simulink library "common_lib"  (R2023a)
settings: Solver=ode45  StartTime=0.0  StopTime=10.0  RelTol=1e-3
undefined symbols (not defined in the file): ACCEL_PRE_MULT, APDT_SrvcMgr_IRVHVDCSubFcnReq, C_C1GearNumbers, C_C1GearRatios, C_Calibration, C_DitherWaveform, C_GearOffset, C_GearRatioIn, C_GearRatioInverseOut, C_GearRatioOut, CLUTCH_INNER_LOOP_UPDATE_RATE, CONSTANT, DEGRADED_MODE_SIZE, Dem_EventStatusType, DiscIntNeverNeededParam, F_FAULT_ENUM, F_NOFAULT, F_OUTOFRANGE, F_RATELIMIT, FALSE, FMI14_SPECIAL_INSTRUCTIONS, FMI20_DATA_DRIFTED_HIGH, FMI21_DATA_DRIFTED_LOW, FMI29_RESERVED_FOR_SAE_ASSIGNMENT, FMI30_RESERVED_FOR_SAE_ASSIGNMENT, FMI31_CONDITION_EXISTS, FMI32_NO_FAULT, IC, k_accel, k_mean, MAX_UINT32, MEAN_PRE_MULT, NTriggers, QLTY_SIGNAL_FAILED, QLTY_SIGNAL_FULLY_FUNCTION, QLTY_SIGNAL_SUBSTITUTED_BY_1ST_CHOICE, QLTY_SIGNAL_SUBSTITUTED_BY_2ND_CHOICE, QLTY_SIGNAL_SUBSTITUTED_BY_3RD_CHOICE, QLTY_SIGNAL_SUBSTITUTED_BY_4TH_CHOICE, SAMPLE_TIME_100us, SAMPLETIME_10ms_Int, SATURATION_U16, simin, T_TestPoint, TF_FALSE, TF_TRUE, TimeStep, TRUE, WORKSPACE_UPDATE_RATE, ZERO, Zero
libraries: $bdroot x123, simulink x28, simulink_extras x4, MBD_EPS_Local_Blockset x4
(part 4 of 10)

== system common_lib/Approved Simulink/Basic IO ==
  note: HWin/ HWout
  note: Product Test
  note: Data Monitor, VPA, SnapShot
  Inport : Inport
  C_Calibration : $bdroot/IO/Calibration with Pretty Print Value  CalValue=C_Calibration  scaling=None
  Constant : Constant  Value=CONSTANT  SampleTime=-1
  DRDataStoreRead : DataStoreRead  DataStoreName=DataStoreRead  SampleTime=0  IndexOptions=Index vector (dialog)  Indices=1  OutputSizes=1
  DRDataStoreRead1 : DataStoreRead  DataStoreName=PT_ProductTest_Read  SampleTime=0  IndexOptions=Index vector (dialog)  Indices=1  OutputSizes=1
  DRDataStoreRead2 : DataStoreRead  DataStoreName=DM_DataMonitor_Read  SampleTime=0  IndexOptions=Index vector (dialog)  Indices=1  OutputSizes=1
  DSDataStoreMemory : DataStoreMemory  DataStoreName=DataStoreMemory  ShowAdditionalParam=off
  DSDataStoreMemory1 : DataStoreMemory  DataStoreName=PT_ProductTest_Memory  ShowAdditionalParam=off
  DSDataStoreMemory2 : DataStoreMemory  DataStoreName=DM_DataMonitor  ShowAdditionalParam=off
  DWDataStoreWrite : DataStoreWrite  DataStoreName=DataStoreWrite  IndexOptions=Index vector (dialog)  Indices=1  OutputSizes=1
  DWDataStoreWrite1 : DataStoreWrite  DataStoreName=DataStoreWrite  IndexOptions=Index vector (dialog)  Indices=1  OutputSizes=1
  DWDataStoreWrite2 : DataStoreWrite  DataStoreName=DM_DataMonitor_Write  IndexOptions=Index vector (dialog)  Indices=1  OutputSizes=1
  Ground : Ground
  M_MonitorParameter : ToWorkspace  VariableName=MonitorParameter  SampleTime=WORKSPACE_UPDATE_RATE
      settings: Decimation=WORKSPACE_DECIMATION
  M_MonitorParameter1 : Subsystem  mask{work=ToWorkspace}
      mask prompts: work "Variable Name"
      mask init:
      | set_param([gcb,'/towork'],'VariableName',work);
      | a = get_param([gcb '/Input'],'LineHandles');
      | set(a.Outport,'Name',work)
      mask Display:
      | patch([.01 .01 .99 .99],[.01 .99 .99 .01],[0 .8 0])
      | disp(work)
  T_TestPoint : Constant  Value=T_TestPoint  SampleTime=-1
  Terminator : Terminator
  To xPC Scope1 : Subsystem  mask(To Workspace Simulation){UserName=, SampleRate=-1, Prio=Low, NameFromSignal=on}
      mask prompts: UserName "Name"; SampleRate "Sample Rate"; Prio "Priority"; NameFromSignal "Name From Signal"
      mask help:
      | "Green Blocks" will record signals during simulation. The Name is now
      | required to come from the signal name so the "Name From Signal" box should
      | be checked. Please select the appropriate Priority Level to ensure optimal
      | simulation runtime and resource use.
      |
      | High - Will ALWAYS record. Choose this if it is a critical signal that
      |        everyone would benefit from having.
      |
      | Med  - A signal that is important to a particular subsystem for testing
      |        purposes. If testing that subsystem you will likely desire this
      |        signal
      |
      | Low  - For debug purposes within a subsystem. This is for obtaining maximum
      |        information in a subsystem to understand every step of logic during
      |        simulation
      mask init:
      | myPrio = 0;
      | sigName = '';
      | 
      | switch (Prio)
      |     case 'Low'
      |         myPrio = 3;
      |     case 'Med'
      |         myPrio = 2;
      |     case 'High'
      |         myPrio = 1;
      | end
      | 
      | if NameFromSignal || isempty(UserName)
      |     sigName = get_param(gcb, 'InputSignalNames');   % Get the name of the signal
      |     sigName = regexprep(sigName{1}, '[<> ]', '');
      | else
      |     sigName = UserName;
      | end
      | 
      | if ~isempty(sigName)
      |     if myPrio <= getPriority(char(gcb))
      |         tmLst = find_system(gcb, 'FollowLinks', 'on', 'LookUnderMasks', 'on', 'BlockType', 'Terminator');
      |         if ~isempty(tmLst)
      |             pos = get_param(tmLst{1}, 'Position');
      |             delete_block(tmLst{1});
      |             newPos = [pos(1), pos(2), pos(1) + 85, pos(2) + 20];
      |             add_block('built-in/ToWorkspace', [char(gcb) '/ToWorkspace'], ...
      |                 'Position', newPos, ...
      |                 'VariableName', ['SIMOUT_' char(sigName)], ...
      |                 'SampleTime', '-1', ...
      |                 'SaveFormat', 'Structure With Time', ...
      |                 'MaxDataPoints', 'Inf');
      |         end
      |     else
      |         twsLst = find_system(gcb, 'FollowLinks', 'on', 'LookUnderMasks', 'on', 'BlockType', 'ToWorkspace');
      |         if ~isempty(twsLst)
      |             pos = get_param(twsLst{1}, 'Position');
      |             delete_block(twsLst{1});
      |             newPos = [pos(1), pos(2), pos(1) + 20, pos(2) + 20];
      |             add_block('built-in/Terminator', [char(gcb) '/Terminate'], 'Position', newPos);
      |         end
      |     end
      | end
      mask TypeOptions Prio: Low | Med | High
      mask Display: disp(Prio)
  Outport : Outport  VectorParamsAs1DForOutWhenUnconnected=off

== system common_lib/Approved Simulink/Discrete And Discontinuities ==
  Dead Zone Dynamic : simulink/Discontinuities/Dead Zone Dynamic
  Discrete-Time Integrator : DiscreteIntegrator  ICPrevOutput=DiscIntNeverNeededParam  ICPrevScaledInput=DiscIntNeverNeededParam
  Rate Limiter : RateLimiter  SampleTimeMode=inherited
  Relay : Relay
  Saturation : Saturate
  Saturation Dynamic : simulink/Discontinuities/Saturation Dynamic  OutMin=[]  OutMax=[]  OutDataTypeStr=Inherit: Same as second input  OutDataType=fixdt(1, 16)  OutScaling=2^-10  DoSatur=off
  Unit Delay : UnitDelay  InitialCondition=IC  SampleTime=-1  HasFrameUpgradeWarning=on
      settings: AttributesFormatString=ic=%<X0>
  Zero-Order Hold : ZeroOrderHold

== system common_lib/Approved Simulink/Flip Flops ==
  D Flip-Flop : simulink_extras/Flip Flops/D Flip-Flop
  D Latch : simulink_extras/Flip Flops/D Latch
  J-K Flip-Flop : simulink_extras/Flip Flops/J-K Flip-Flop  initial_condition=0
  S-R Flip-Flop : simulink_extras/Flip Flops/S-R Flip-Flop  initial_condition=0

== system common_lib/Approved Simulink/Grouping ==
  note: Busses are preferred to
      | MUXes except where array definition
      | or linear algebra requires a MUX
  Bus Creator : BusCreator  Inputs=2
  Bus Selector : BusSelector  OutputSignals=signal1,signal2
  Demux : Demux  Outputs=2
  Merge : Merge
  Mux : Mux  Inputs=2
  Selector : Selector  InputPortWidth=3  IndexOptions=Index vector (dialog)  Indices=[1 3]  OutputSizes=1

== system common_lib/Approved Simulink/Math And Logic ==
  Abs : Abs  ZeroCross=off  SaturateOnIntegerOverflow=off
  Assignment : Assignment  IndexOptions=Index vector (dialog)  Indices=1  OutputSizes=1
  Gain : Gain
  Logical Operator : Logic  Operator=OR  AllPortsSameDT=off
  Math Function : Math  SignedPower=on
  MinMax : MinMax  Inputs=2  InputSameDT=on  ZeroCross=off
  Multiport Switch : MultiPortSwitch  SaturateOnIntegerOverflow=off  InputSameDT=off
  Product1 : Product  OutDataTypeStr=Inherit: Same as first input
  Relational Operator : RelationalOperator  Operator=<=  ZeroCross=off  InputSameDT=off
  Sign : Signum
  Sum : Sum  Inputs=|+-
  Switch : Switch  Threshold=0.5  ZeroCross=off  SaturateOnIntegerOverflow=off  InputSameDT=off

== system common_lib/Approved Simulink/Signal Attributes ==
  Data Type Conversion : DataTypeConversion  SaturateOnIntegerOverflow=off
  Rate Transition : RateTransition
  Signal Conversion : SignalConversion  ConversionOutput=Contiguous copy  OverrideOpt=off

== system common_lib/Approved Simulink/SubSys Triggers ==
  Enable : EnablePort  ZeroCross=off
  Trigger : TriggerPort  VariantControl=(inherit)  ZeroCross=off
  Configurable Subsystem : Subsystem
      settings: TemplateBlock=self
  For Iterator Subsystem : Subsystem  TreatAsAtomicUnit=on
  Function-Call Generator : simulink/Ports & Subsystems/Function-Call Generator  sample_time=1  numberOfIterations=1  DisallowWideOutput=off
  If : If
  If Action Subsystem : Subsystem  TreatAsAtomicUnit=on
  Subsystem : Subsystem
  Switch Case : SwitchCase
  While Iterator Subsystem : Subsystem  TreatAsAtomicUnit=on

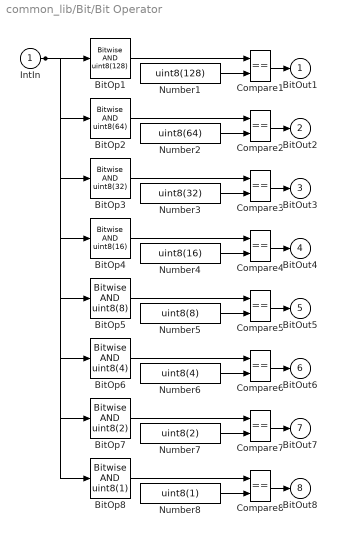
== system common_lib/Bit/Bit Operator ==
  IntIn : Inport
  BitOp1 : simulink/Logic and Bit Operations/Bitwise Operator  logicop=AND  UseBitMask=on  BitMask=uint8(128)  BitMaskRealWorld=Stored Integer
  BitOp2 : simulink/Logic and Bit Operations/Bitwise Operator  logicop=AND  UseBitMask=on  BitMask=uint8(64)  BitMaskRealWorld=Stored Integer
  BitOp3 : simulink/Logic and Bit Operations/Bitwise Operator  logicop=AND  UseBitMask=on  BitMask=uint8(32)  BitMaskRealWorld=Stored Integer
  BitOp4 : simulink/Logic and Bit Operations/Bitwise Operator  logicop=AND  UseBitMask=on  BitMask=uint8(16)  BitMaskRealWorld=Stored Integer
  BitOp5 : simulink/Logic and Bit Operations/Bitwise Operator  logicop=AND  UseBitMask=on  BitMask=uint8(8)  BitMaskRealWorld=Stored Integer
  BitOp6 : simulink/Logic and Bit Operations/Bitwise Operator  logicop=AND  UseBitMask=on  BitMask=uint8(4)  BitMaskRealWorld=Stored Integer
  BitOp7 : simulink/Logic and Bit Operations/Bitwise Operator  logicop=AND  UseBitMask=on  BitMask=uint8(2)  BitMaskRealWorld=Stored Integer
  BitOp8 : simulink/Logic and Bit Operations/Bitwise Operator  logicop=AND  UseBitMask=on  BitMask=uint8(1)  BitMaskRealWorld=Stored Integer
  Compare{1..8} (8 alike) : RelationalOperator  Operator===
  Number1 : Constant  Value=uint8(128)
  Number2 : Constant  Value=uint8(64)
  Number3 : Constant  Value=uint8(32)
  Number4 : Constant  Value=uint8(16)
  Number5 : Constant  Value=uint8(8)
  Number6 : Constant  Value=uint8(4)
  Number7 : Constant  Value=uint8(2)
  Number8 : Constant  Value=uint8(1)
  BitOut1 : Outport  VectorParamsAs1DForOutWhenUnconnected=off
  BitOut2 : Outport  Port=2  VectorParamsAs1DForOutWhenUnconnected=off
  BitOut3 : Outport  Port=3  VectorParamsAs1DForOutWhenUnconnected=off
  BitOut4 : Outport  Port=4  VectorParamsAs1DForOutWhenUnconnected=off
  BitOut5 : Outport  Port=5  VectorParamsAs1DForOutWhenUnconnected=off
  BitOut6 : Outport  Port=6  VectorParamsAs1DForOutWhenUnconnected=off
  BitOut7 : Outport  Port=7  VectorParamsAs1DForOutWhenUnconnected=off
  BitOut8 : Outport  Port=8  VectorParamsAs1DForOutWhenUnconnected=off
  wires:
  BitOp1/1 -> Compare1/1
  Number1/1 -> Compare1/2
  Compare1/1 -> BitOut1/1
  IntIn/1 -> BitOp1/1, BitOp2/1, BitOp3/1, BitOp4/1, BitOp5/1, BitOp6/1, BitOp7/1, BitOp8/1
  BitOp2/1 -> Compare2/1
  Number2/1 -> Compare2/2
  Compare2/1 -> BitOut2/1
  BitOp3/1 -> Compare3/1
  Number3/1 -> Compare3/2
  Compare3/1 -> BitOut3/1
  BitOp4/1 -> Compare4/1
  Number4/1 -> Compare4/2
  Compare4/1 -> BitOut4/1
  BitOp5/1 -> Compare5/1
  Number5/1 -> Compare5/2
  Compare5/1 -> BitOut5/1
  BitOp6/1 -> Compare6/1
  Number6/1 -> Compare6/2
  Compare6/1 -> BitOut6/1
  BitOp7/1 -> Compare7/1
  Number7/1 -> Compare7/2
  Compare7/1 -> BitOut7/1
  BitOp8/1 -> Compare8/1
  Number8/1 -> Compare8/2
  Compare8/1 -> BitOut8/1

== system common_lib/Ctrl/Derivative ==
  note: Common Library::Derivative
  input : Inport
  cutoff : Inport  Port=2
  ulim : Inport  Port=3
  llim : Inport  Port=4
  reset? : Inport  Port=5  OutDataTypeStr=boolean
  Data Type Conversion : DataTypeConversion  OutDataTypeStr=boolean  SaturateOnIntegerOverflow=off  RndMeth=Floor
  Data Type Conversion1 : DataTypeConversion  OutDataTypeStr=single  SaturateOnIntegerOverflow=off  RndMeth=Floor
  Data Type Conversion2 : DataTypeConversion  OutDataTypeStr=single  SaturateOnIntegerOverflow=off  RndMeth=Floor
  DerivativeCoreLogic : Subsystem  TreatAsAtomicUnit=on  RTWFcnName=DER
      settings: RTWFcnNameOpts=User specified  RTWFileNameOpts=Use function name
  Gain : Gain  Gain=Ts
  Product1 : Product  Inputs=**  InputSameDT=on  OutDataTypeStr=Inherit: Same as first input
  Signal Conversion : SignalConversion  ConversionOutput=Contiguous copy  OverrideOpt=off
  output : Outport  VectorParamsAs1DForOutWhenUnconnected=off
  wires:
  input/1 -> Product1/1
  cutoff/1 -> Product1/2, Gain/1
  DerivativeCoreLogic/1(output) -> Signal Conversion/1
  reset?/1 -> Data Type Conversion/1
  Gain/1 -> DerivativeCoreLogic/2(cutoff)
  Product1/1 -> DerivativeCoreLogic/1(input)
  ulim/1 -> Data Type Conversion1/1
  llim/1 -> Data Type Conversion2/1
  Data Type Conversion/1 -> DerivativeCoreLogic/3(reset?)
  Data Type Conversion1/1 -> DerivativeCoreLogic/4(ulim)
  Data Type Conversion2/1 -> DerivativeCoreLogic/5(llim)
  Signal Conversion/1 -> output/1

== system common_lib/Ctrl/Dither ==
  note: Filter output waveform to smooth
      | the transitions if necessary.
  note: Keep present output state until
      | number of executions has occured.
      | (initialize to FALSE)
  note: Keep track of number of iterations
      | since last output transition.
      | (initialize to zero)
  note: Calculate number of executions
      | between alternating output.
      | 1/ (2 * TimeStep * frequency)
      | Add in half a frame to roundoff to
      | nearest minor frame boundary
  note: Simple Dither Function
      | Outputs a modified rectangular wave of specified
      | amplitude, frequency and filter constant.
  note: Common Library::Dither
  amplitude : Inport
  frequency : Inport  Port=2
  tau : Inport  Port=3
  Constant1 : Constant  Value=MinusOne
  Constant14 : Constant  Value=int16(1)
  Constant2 : Constant  Value=One
  Constant3 : Constant  Value=Two
  Constant4 : Constant  Value=One
  Constant5 : Constant  Value=lim
  Constant6 : Constant  Value=One
  Constant7 : Constant  Value=int16(1)
  Constant8 : Constant  Value=TimeStep
  Constant9 : Constant  Value=ZeroFive
  Data Type Conversion : DataTypeConversion  OutDataTypeStr=single  SaturateOnIntegerOverflow=off
  Data Type Conversion1 : DataTypeConversion  OutDataTypeStr=single  SaturateOnIntegerOverflow=off  RndMeth=Floor
  Fltr : $bdroot/Fltrs/Fltr  TimeStep=TimeStep
  Logical Operator : Logic  Operator=NOT
  MinMax1 : MinMax  Inputs=2  InputSameDT=on  SaturateOnIntegerOverflow=on  ZeroCross=off
  MinMax2 : MinMax  Function=max  Inputs=2  InputSameDT=on  SaturateOnIntegerOverflow=on  ZeroCross=off
  Product1 : Product  Inputs=**  InputSameDT=on  OutDataTypeStr=Inherit: Same as first input
  Product2 : Product  Inputs=***  InputSameDT=on  OutDataTypeStr=Inherit: Same as first input
  Product3 : Product  Inputs=*/  InputSameDT=on  OutDataTypeStr=Inherit: Same as first input
  Relational Operator : RelationalOperator  Operator=<  ZeroCross=off
  Sum1 : Sum  Inputs=|++  InputSameDT=on  OutDataTypeStr=Inherit: Same as first input
  Sum3 : Sum  Inputs=++|  InputSameDT=on  OutDataTypeStr=Inherit: Same as first input
  Switch1 : Switch  Threshold=0.5  ZeroCross=off  SaturateOnIntegerOverflow=off
  Switch2 : Switch  Threshold=0.5  ZeroCross=off  SaturateOnIntegerOverflow=off
  Switch3 : Switch  Threshold=0.5  ZeroCross=off  SaturateOnIntegerOverflow=off
  Unit Delay1 : UnitDelay  InitialCondition=int16(0)  SampleTime=-1  HasFrameUpgradeWarning=on
  Unit Delay11 : UnitDelay  InitialCondition=false  SampleTime=-1  HasFrameUpgradeWarning=on
  output : Outport  VectorParamsAs1DForOutWhenUnconnected=off
  wires:
  Constant8/1 -> Data Type Conversion1/1
  Data Type Conversion1/1 -> Product2/1
  Constant9/1 -> Sum1/2
  Sum1/1 -> Relational Operator/2
  Data Type Conversion/1 -> Relational Operator/1
  Relational Operator/1 -> Switch1/2, Switch3/2
  Product3/1 -> Sum1/1
  Logical Operator/1 -> Switch1/3
  Sum3/1 -> Data Type Conversion/1, Switch3/1
  Constant7/1 -> Sum3/1
  Unit Delay1/1 -> Sum3/2
  Constant14/1 -> Switch3/3
  Switch3/1 -> Unit Delay1/1
  Constant3/1 -> Product2/3
  Constant6/1 -> Product3/1
  MinMax2/1 -> Product3/2
  Fltr/1 -> output/1
  Constant5/1 -> MinMax2/2
  MinMax1/1 -> MinMax2/1
  Constant4/1 -> MinMax1/2
  Product2/1 -> MinMax1/1
  frequency/1 -> Product2/2
  amplitude/1 -> Product1/1
  Switch2/1 -> Product1/2
  Constant2/1 -> Switch2/1
  Constant1/1 -> Switch2/3
  Product1/1 -> Fltr/1
  Switch1/1 -> Switch2/2, Unit Delay11/1
  Unit Delay11/1 -> Switch1/1, Logical Operator/1
  tau/1 -> Fltr/2

== system common_lib/Ctrl/Dither w Reset ==
  note: Filter output waveform to smooth
      | the transitions if necessary.
  note: Keep present output state until
      | number of executions has occured.
      | (initialize to FALSE)
  note: Keep track of number of iterations
      | since last output transition.
      | (initialize to zero)
  note: Calculate number of executions
      | between alternating output.
      | 1/ (2 * TimeStep * frequency)
      | Add in half a frame to roundoff to
      | nearest minor frame boundary
  note: Simple Dither Function
      | Outputs a modified rectangular wave of specified
      | amplitude, frequency and filter constant.  Also
      | provides a reset signal on switch of output sign.
  note: Common Library::Dither with Reset
  amplitude : Inport
  frequency : Inport  Port=2
  tau : Inport  Port=3
  Constant1 : Constant  Value=MinusOne
  Constant14 : Constant  Value=int16(1)
  Constant2 : Constant  Value=One
  Constant3 : Constant  Value=Two
  Constant4 : Constant  Value=One
  Constant5 : Constant  Value=lim
  Constant6 : Constant  Value=One
  Constant7 : Constant  Value=int16(1)
  Constant8 : Constant  Value=TimeStep
  Constant9 : Constant  Value=ZeroFive
  Data Type Conversion : DataTypeConversion  OutDataTypeStr=single  SaturateOnIntegerOverflow=off
  Data Type Conversion1 : DataTypeConversion  OutDataTypeStr=single  SaturateOnIntegerOverflow=off  RndMeth=Floor
  Fltr : $bdroot/Fltrs/Fltr  TimeStep=TimeStep
  Logical Operator : Logic  Operator=NOT
  Logical Operator1 : Logic  Operator=NOT
  MinMax1 : MinMax  Inputs=2  InputSameDT=on  SaturateOnIntegerOverflow=on  ZeroCross=off
  MinMax2 : MinMax  Function=max  Inputs=2  InputSameDT=on  SaturateOnIntegerOverflow=on  ZeroCross=off
  Product1 : Product  Inputs=**  InputSameDT=on  OutDataTypeStr=Inherit: Same as first input
  Product2 : Product  Inputs=***  InputSameDT=on  OutDataTypeStr=Inherit: Same as first input
  Product3 : Product  Inputs=*/  InputSameDT=on  OutDataTypeStr=Inherit: Same as first input
  Relational Operator : RelationalOperator  Operator=<  ZeroCross=off
  Sum1 : Sum  Inputs=|++  InputSameDT=on  OutDataTypeStr=Inherit: Same as first input
  Sum3 : Sum  Inputs=++|  InputSameDT=on  OutDataTypeStr=Inherit: Same as first input
  Switch1 : Switch  Threshold=0.5  ZeroCross=off  SaturateOnIntegerOverflow=off
  Switch2 : Switch  Threshold=0.5  ZeroCross=off  SaturateOnIntegerOverflow=off
  Switch3 : Switch  Threshold=0.5  ZeroCross=off  SaturateOnIntegerOverflow=off
  Unit Delay1 : UnitDelay  InitialCondition=int16(0)  SampleTime=-1  HasFrameUpgradeWarning=on
  Unit Delay11 : UnitDelay  InitialCondition=false  SampleTime=-1  HasFrameUpgradeWarning=on
  output : Outport  VectorParamsAs1DForOutWhenUnconnected=off
  reset : Outport  Port=2  VectorParamsAs1DForOutWhenUnconnected=off
  wires:
  Constant8/1 -> Data Type Conversion1/1
  Data Type Conversion1/1 -> Product2/1
  Constant9/1 -> Sum1/2
  Sum1/1 -> Relational Operator/2
  Data Type Conversion/1 -> Relational Operator/1
  Relational Operator/1 -> Logical Operator1/1, Switch1/2, Switch3/2
  Product3/1 -> Sum1/1
  Logical Operator/1 -> Switch1/3
  Sum3/1 -> Data Type Conversion/1, Switch3/1
  Constant7/1 -> Sum3/1
  Unit Delay1/1 -> Sum3/2
  Constant14/1 -> Switch3/3
  Switch3/1 -> Unit Delay1/1
  Constant3/1 -> Product2/3
  Constant6/1 -> Product3/1
  MinMax2/1 -> Product3/2
  Fltr/1 -> output/1
  Constant5/1 -> MinMax2/2
  MinMax1/1 -> MinMax2/1
  Constant4/1 -> MinMax1/2
  Product2/1 -> MinMax1/1
  frequency/1 -> Product2/2
  amplitude/1 -> Product1/1
  Switch2/1 -> Product1/2
  Constant2/1 -> Switch2/1
  Constant1/1 -> Switch2/3
  Product1/1 -> Fltr/1
  Switch1/1 -> Switch2/2, Unit Delay11/1
  Unit Delay11/1 -> Switch1/1, Logical Operator/1
  tau/1 -> Fltr/2
  Logical Operator1/1 -> reset/1

== system common_lib/Ctrl/Integrator ==
  note: Common Library::Integral
  input : Inport
  ulim : Inport  Port=2
  llim : Inport  Port=3
  ic : Inport  Port=4
  reset? : Inport  Port=5  OutDataTypeStr=boolean
  Constant1 : Constant  Value=TimeStep
  Data Type Conversion : DataTypeConversion  OutDataTypeStr=single  RndMeth=Floor
  Product1 : Product  Inputs=**  InputSameDT=on  SaturateOnIntegerOverflow=on  OutDataTypeStr=Inherit: Same as first input
  Sat : $bdroot/Slink/Sat
  Sum : Sum  Inputs=++|  InputSameDT=on  SaturateOnIntegerOverflow=on  OutDataTypeStr=Inherit: Same as first input
  Switch : Switch  Threshold=0.5  ZeroCross=off
  Unit Delay : UnitDelay  InitialCondition=IC  SampleTime=-1  HasFrameUpgradeWarning=on
  Output : Outport  VectorParamsAs1DForOutWhenUnconnected=off
  wires:
  Constant1/1 -> Data Type Conversion/1
  Data Type Conversion/1 -> Product1/1
  Sat/1 -> Unit Delay/1, Output/1
  Unit Delay/1 -> Sum/1
  Switch/1 -> Sat/1
  Sum/1 -> Switch/3
  llim/1 -> Sat/3
  ulim/1 -> Sat/2
  reset?/1 -> Switch/2
  Product1/1 -> Sum/2
  ic/1 -> Switch/1
  input/1 -> Product1/2

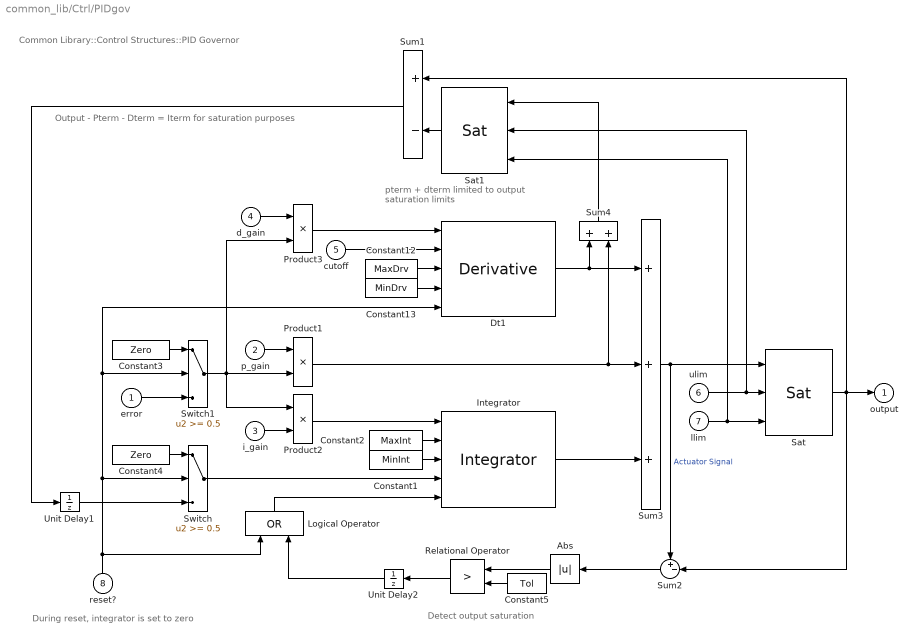
== system common_lib/Ctrl/PIDgov ==
  note: pterm + dterm
      | limited to output saturation limits
  note: Common Library::Control Structures::PID Governor
  note: Detect output saturation
  note: Output - Pterm - Dterm = Iterm for saturation purposes
  note: During reset, integrator is set to zero
  error : Inport
  p_gain : Inport  Port=2
  i_gain : Inport  Port=3
  d_gain : Inport  Port=4
  cutoff : Inport  Port=5
  ulim : Inport  Port=6
  llim : Inport  Port=7
  reset? : Inport  Port=8  OutDataTypeStr=boolean
  Abs : Abs  ZeroCross=off  SaturateOnIntegerOverflow=off
  Constant1 : Constant  Value=MinInt
  Constant12 : Constant  Value=MaxDrv
  Constant13 : Constant  Value=MinDrv
  Constant2 : Constant  Value=MaxInt
  Constant3 : Constant  Value=Zero
  Constant4 : Constant  Value=Zero
  Constant5 : Constant  Value=Tol
  Dt1 : $bdroot/Ctrl/Derivative  TimeStep=TimeStep
  Integrator : $bdroot/Ctrl/Integrator  TimeStep=TimeStep  IC=IC
  Logical Operator : Logic  Operator=OR
  Product1 : Product  InputSameDT=on  OutDataTypeStr=Inherit: Same as first input
  Product2 : Product  InputSameDT=on  OutDataTypeStr=Inherit: Same as first input
  Product3 : Product  InputSameDT=on  OutDataTypeStr=Inherit: Same as first input
  Relational Operator : RelationalOperator  Operator=>  ZeroCross=off
  Sat : $bdroot/Slink/Sat
  Sat1 : $bdroot/Slink/Sat
  Sum1 : Sum  Inputs=+-  InputSameDT=on  OutDataTypeStr=Inherit: Same as first input
  Sum2 : Sum  Inputs=+-|  InputSameDT=on  OutDataTypeStr=Inherit: Same as first input
  Sum3 : Sum  Inputs=+++  InputSameDT=on  OutDataTypeStr=Inherit: Same as first input
  Sum4 : Sum  InputSameDT=on  OutDataTypeStr=Inherit: Same as first input
  Switch : Switch  Threshold=0.5  ZeroCross=off  SaturateOnIntegerOverflow=off
  Switch1 : Switch  Threshold=0.5  ZeroCross=off  SaturateOnIntegerOverflow=off
  Unit Delay1 : UnitDelay  InitialCondition=Zero  SampleTime=-1  HasFrameUpgradeWarning=on
      settings: AttributesFormatString=ic=%<X0>
  Unit Delay2 : UnitDelay  InitialCondition=false  SampleTime=-1  HasFrameUpgradeWarning=on
      settings: AttributesFormatString=ic=%<X0>
  output : Outport  InitialOutput=8.973  VectorParamsAs1DForOutWhenUnconnected=off
  wires:
  Switch1/1 -> Product1/2, Product2/1, Product3/2
  error/1 -> Switch1/3
  Constant3/1 -> Switch1/1
  cutoff/1 -> Dt1/2
  Constant12/1 -> Dt1/3
  Constant13/1 -> Dt1/4
  Sat1/1 -> Sum1/2
  Sum4/1 -> Sat1/1
  Dt1/1 -> Sum3/1, Sum4/1
  Unit Delay1/1 -> Switch/3
  Sum2/1 -> Abs/1
  Relational Operator/1 -> Unit Delay2/1
  Abs/1 -> Relational Operator/1
  Constant5/1 -> Relational Operator/2
  Constant2/1 -> Integrator/2
  Constant1/1 -> Integrator/3
  reset?/1 -> Switch1/2, Dt1/5, Switch/2, Logical Operator/1
  ulim/1 -> Sat1/2, Sat/2
  p_gain/1 -> Product1/1
  Product1/1 -> Sum3/2, Sum4/2
  llim/1 -> Sat1/3, Sat/3
  Sum3/1 -> Sat/1, Sum2/1  "Actuator Signal"
  Sat/1 -> Sum1/1, output/1, Sum2/2
  i_gain/1 -> Product2/2
  Constant4/1 -> Switch/1
  Logical Operator/1 -> Integrator/5
  Unit Delay2/1 -> Logical Operator/2
  Switch/1 -> Integrator/4
  Integrator/1 -> Sum3/3
  Sum1/1 -> Unit Delay1/1
  Product2/1 -> Integrator/1
  Product3/1 -> Dt1/1
  d_gain/1 -> Product3/1

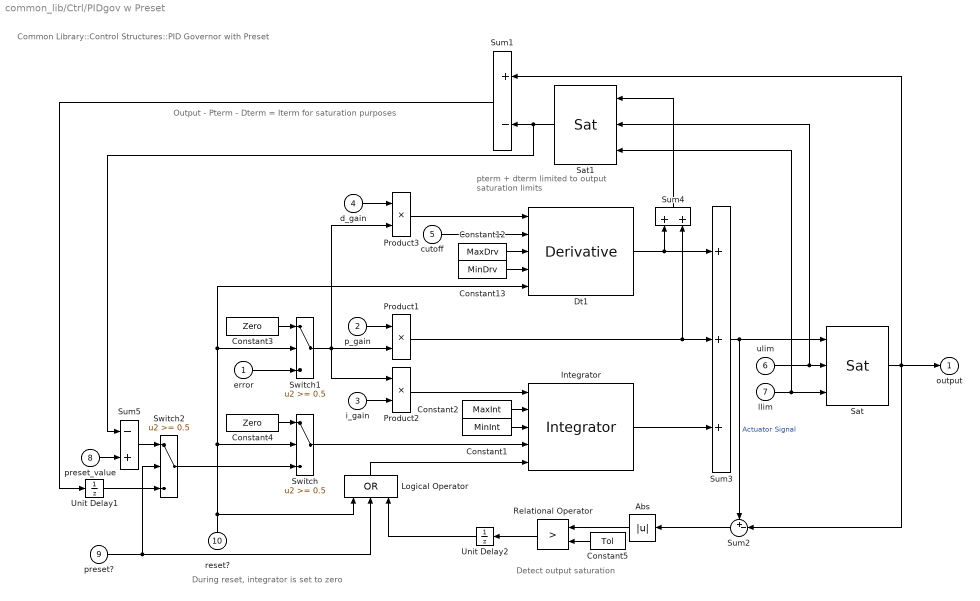
== system common_lib/Ctrl/PIDgov w Preset ==
  note: pterm + dterm
      | limited to output saturation limits
  note: Common Library::Control Structures::PID Governor with Preset
  note: Detect output saturation
  note: Output - Pterm - Dterm = Iterm for saturation purposes
  note: During reset, integrator is set to zero
  error : Inport
  p_gain : Inport  Port=2
  i_gain : Inport  Port=3
  d_gain : Inport  Port=4
  cutoff : Inport  Port=5
  ulim : Inport  Port=6
  llim : Inport  Port=7
  preset_value : Inport  Port=8
  preset? : Inport  Port=9
  reset? : Inport  Port=10  OutDataTypeStr=boolean
  Abs : Abs  ZeroCross=off  SaturateOnIntegerOverflow=off
  Constant1 : Constant  Value=MinInt
  Constant12 : Constant  Value=MaxDrv
  Constant13 : Constant  Value=MinDrv
  Constant2 : Constant  Value=MaxInt
  Constant3 : Constant  Value=Zero
  Constant4 : Constant  Value=Zero
  Constant5 : Constant  Value=Tol
  Dt1 : $bdroot/Ctrl/Derivative  TimeStep=TimeStep
  Integrator : $bdroot/Ctrl/Integrator  TimeStep=TimeStep  IC=IC
  Logical Operator : Logic  Operator=OR  Inputs=3
  Product1 : Product  InputSameDT=on  OutDataTypeStr=Inherit: Same as first input
  Product2 : Product  InputSameDT=on  OutDataTypeStr=Inherit: Same as first input
  Product3 : Product  InputSameDT=on  OutDataTypeStr=Inherit: Same as first input
  Relational Operator : RelationalOperator  Operator=>  ZeroCross=off
  Sat : $bdroot/Slink/Sat
  Sat1 : $bdroot/Slink/Sat
  Sum1 : Sum  Inputs=+-  InputSameDT=on  OutDataTypeStr=Inherit: Same as first input
  Sum2 : Sum  Inputs=+-|  InputSameDT=on  OutDataTypeStr=Inherit: Same as first input
  Sum3 : Sum  Inputs=+++  InputSameDT=on  OutDataTypeStr=Inherit: Same as first input
  Sum4 : Sum  InputSameDT=on  OutDataTypeStr=Inherit: Same as first input
  Sum5 : Sum  Inputs=-+  InputSameDT=on  OutDataTypeStr=Inherit: Same as first input
  Switch : Switch  Threshold=0.5  ZeroCross=off  SaturateOnIntegerOverflow=off
  Switch1 : Switch  Threshold=0.5  ZeroCross=off  SaturateOnIntegerOverflow=off
  Switch2 : Switch  Threshold=0.5  ZeroCross=off  SaturateOnIntegerOverflow=off
  Unit Delay1 : UnitDelay  InitialCondition=Zero  SampleTime=-1  HasFrameUpgradeWarning=on
      settings: AttributesFormatString=ic=%<X0>
  Unit Delay2 : UnitDelay  InitialCondition=false  SampleTime=-1  HasFrameUpgradeWarning=on
      settings: AttributesFormatString=ic=%<X0>
  output : Outport  InitialOutput=8.973  VectorParamsAs1DForOutWhenUnconnected=off
  wires:
  Sum5/1 -> Switch2/1
  preset_value/1 -> Sum5/2
  Switch2/1 -> Switch/3
  Unit Delay1/1 -> Switch2/3
  Switch1/1 -> Product1/2, Product2/1, Product3/2
  error/1 -> Switch1/3
  Constant3/1 -> Switch1/1
  cutoff/1 -> Dt1/2
  Constant12/1 -> Dt1/3
  Constant13/1 -> Dt1/4
  preset?/1 -> Switch2/2, Logical Operator/2
  Sat1/1 -> Sum5/1, Sum1/2
  Sum4/1 -> Sat1/1
  Dt1/1 -> Sum3/1, Sum4/1
  Sum2/1 -> Abs/1
  Relational Operator/1 -> Unit Delay2/1
  Abs/1 -> Relational Operator/1
  Constant5/1 -> Relational Operator/2
  Constant2/1 -> Integrator/2
  Constant1/1 -> Integrator/3
  reset?/1 -> Switch1/2, Dt1/5, Switch/2, Logical Operator/1
  ulim/1 -> Sat1/2, Sat/2
  p_gain/1 -> Product1/1
  Product1/1 -> Sum3/2, Sum4/2
  llim/1 -> Sat1/3, Sat/3
  Sum3/1 -> Sat/1, Sum2/1  "Actuator Signal"
  Sat/1 -> Sum1/1, output/1, Sum2/2
  i_gain/1 -> Product2/2
  Constant4/1 -> Switch/1
  Logical Operator/1 -> Integrator/5
  Unit Delay2/1 -> Logical Operator/3
  Switch/1 -> Integrator/4
  Integrator/1 -> Sum3/3
  Sum1/1 -> Unit Delay1/1
  Product2/1 -> Integrator/1
  Product3/1 -> Dt1/1
  d_gain/1 -> Product3/1

== system common_lib/Ctrl/PIgov ==
  note: pterm
      | limited to output saturation limits
  note: Common Library::Control Structures::PI Governor
  note: Detect output saturation
  note: Output - Pterm - Dterm = Iterm for saturation purposes
  note: During reset, integrator is set to zero
  error : Inport
  p_gain : Inport  Port=2
  i_gain : Inport  Port=3
  ulim : Inport  Port=4
  llim : Inport  Port=5
  reset? : Inport  Port=6  OutDataTypeStr=boolean
  Abs : Abs  ZeroCross=off
  Constant1 : Constant  Value=MinInt
  Constant2 : Constant  Value=MaxInt
  Constant3 : Constant  Value=Zero
  Constant4 : Constant  Value=Zero
  Constant5 : Constant  Value=Tol
  Integrator : $bdroot/Ctrl/Integrator  TimeStep=TimeStep  IC=IC
  Logical Operator : Logic  Operator=OR
  Product1 : Product  InputSameDT=on  SaturateOnIntegerOverflow=on  OutDataTypeStr=Inherit: Same as first input
  Product2 : Product  InputSameDT=on  SaturateOnIntegerOverflow=on  OutDataTypeStr=Inherit: Same as first input
  Relational Operator : RelationalOperator  Operator=>  ZeroCross=off
  Sat : $bdroot/Slink/Sat
  Sat1 : $bdroot/Slink/Sat
  Sum1 : Sum  Inputs=+-  InputSameDT=on  SaturateOnIntegerOverflow=on  OutDataTypeStr=Inherit: Same as first input
  Sum2 : Sum  Inputs=+-|  InputSameDT=on  SaturateOnIntegerOverflow=on  OutDataTypeStr=Inherit: Same as first input
  Sum3 : Sum  InputSameDT=on  SaturateOnIntegerOverflow=on  OutDataTypeStr=Inherit: Same as first input
  Switch : Switch  Threshold=0.5  ZeroCross=off
  Switch1 : Switch  Threshold=0.5  ZeroCross=off
  Unit Delay1 : UnitDelay  InitialCondition=Zero  SampleTime=-1  HasFrameUpgradeWarning=on
      settings: AttributesFormatString=ic=%<X0>
  Unit Delay2 : UnitDelay  InitialCondition=false  SampleTime=-1  HasFrameUpgradeWarning=on
      settings: AttributesFormatString=ic=%<X0>
  output : Outport  InitialOutput=8.973  VectorParamsAs1DForOutWhenUnconnected=off
  wires:
  Switch1/1 -> Product1/2, Product2/1
  error/1 -> Switch1/3
  Constant3/1 -> Switch1/1
  Sat1/1 -> Sum1/2
  Unit Delay1/1 -> Switch/3
  Sum2/1 -> Abs/1
  Relational Operator/1 -> Unit Delay2/1
  Abs/1 -> Relational Operator/1
  Constant5/1 -> Relational Operator/2
  Constant2/1 -> Integrator/2
  Constant1/1 -> Integrator/3
  reset?/1 -> Logical Operator/1, Switch1/2, Switch/2
  ulim/1 -> Sat1/2, Sat/2
  p_gain/1 -> Product1/1
  Product1/1 -> Sum3/1, Sat1/1
  llim/1 -> Sat1/3, Sat/3
  Sum3/1 -> Sat/1, Sum2/1  "Actuator Signal"
  Sat/1 -> Sum1/1, output/1, Sum2/2
  i_gain/1 -> Product2/2
  Constant4/1 -> Switch/1
  Logical Operator/1 -> Integrator/5
  Unit Delay2/1 -> Logical Operator/2
  Switch/1 -> Integrator/4
  Integrator/1 -> Sum3/2
  Sum1/1 -> Unit Delay1/1
  Product2/1 -> Integrator/1

== system common_lib/Ctrl/PIgov w Preset ==
  note: pterm
      | limited to output saturation limits
  note: Common Library::Control Structures::PID Governor with Preset
  note: Detect output saturation
  note: Output - Pterm - Dterm = Iterm for saturation purposes
  note: During reset, integrator is set to zero
  error : Inport
  p_gain : Inport  Port=2
  i_gain : Inport  Port=3
  ulim : Inport  Port=4
  llim : Inport  Port=5
  preset_value : Inport  Port=6
  preset? : Inport  Port=7
  reset? : Inport  Port=8  OutDataTypeStr=boolean
  Abs : Abs  ZeroCross=off  SaturateOnIntegerOverflow=off
  Constant1 : Constant  Value=MinInt
  Constant2 : Constant  Value=MaxInt
  Constant3 : Constant  Value=Zero
  Constant4 : Constant  Value=Zero
  Constant5 : Constant  Value=Tol
  Integrator : $bdroot/Ctrl/Integrator  TimeStep=TimeStep  IC=IC
  Logical Operator : Logic  Operator=OR  Inputs=3
  Product1 : Product  InputSameDT=on  OutDataTypeStr=Inherit: Same as first input
  Product2 : Product  InputSameDT=on  OutDataTypeStr=Inherit: Same as first input
  Relational Operator : RelationalOperator  Operator=>  ZeroCross=off
  Sat : $bdroot/Slink/Sat
  Sat1 : $bdroot/Slink/Sat
  Sum1 : Sum  Inputs=+-  InputSameDT=on  OutDataTypeStr=Inherit: Same as first input
  Sum2 : Sum  Inputs=+-|  InputSameDT=on  OutDataTypeStr=Inherit: Same as first input
  Sum3 : Sum  InputSameDT=on  OutDataTypeStr=Inherit: Same as first input
  Sum4 : Sum  Inputs=-+  InputSameDT=on  OutDataTypeStr=Inherit: Same as first input
  Switch : Switch  Threshold=0.5  ZeroCross=off  SaturateOnIntegerOverflow=off
  Switch1 : Switch  Threshold=0.5  ZeroCross=off  SaturateOnIntegerOverflow=off
  Switch2 : Switch  Threshold=0.5  ZeroCross=off  SaturateOnIntegerOverflow=off
  Unit Delay1 : UnitDelay  InitialCondition=Zero  SampleTime=-1  HasFrameUpgradeWarning=on
      settings: AttributesFormatString=ic=%<X0>
  Unit Delay2 : UnitDelay  InitialCondition=false  SampleTime=-1  HasFrameUpgradeWarning=on
      settings: AttributesFormatString=ic=%<X0>
  output : Outport  InitialOutput=8.973  VectorParamsAs1DForOutWhenUnconnected=off
  wires:
  Sum4/1 -> Switch2/1
  Switch2/1 -> Switch/3
  preset_value/1 -> Sum4/2
  Unit Delay1/1 -> Switch2/3
  Switch1/1 -> Product1/2, Product2/1
  error/1 -> Switch1/3
  Constant3/1 -> Switch1/1
  preset?/1 -> Switch2/2, Logical Operator/2
  Sat1/1 -> Sum4/1, Sum1/2
  Sum2/1 -> Abs/1
  Relational Operator/1 -> Unit Delay2/1
  Abs/1 -> Relational Operator/1
  Constant5/1 -> Relational Operator/2
  Constant2/1 -> Integrator/2
  Constant1/1 -> Integrator/3
  reset?/1 -> Switch1/2, Switch/2, Logical Operator/1
  ulim/1 -> Sat1/2, Sat/2
  p_gain/1 -> Product1/1
  Product1/1 -> Sum3/1, Sat1/1
  llim/1 -> Sat1/3, Sat/3
  Sum3/1 -> Sat/1, Sum2/1  "Actuator Signal"
  Sat/1 -> Sum1/1, output/1, Sum2/2
  i_gain/1 -> Product2/2
  Constant4/1 -> Switch/1
  Logical Operator/1 -> Integrator/5
  Unit Delay2/1 -> Logical Operator/3
  Switch/1 -> Integrator/4
  Integrator/1 -> Sum3/2
  Sum1/1 -> Unit Delay1/1
  Product2/1 -> Integrator/1

== system common_lib/Ctrl/Ramp ==
  note: Common Library::Ramp
  A : Inport
  B : Inport  Port=2
  C : Inport  Port=3
  reset : Inport  Port=4  OutDataTypeStr=boolean
  Constant1 : Constant  Value=TimeStep
  Data Type Conversion : DataTypeConversion  OutDataTypeStr=single  SaturateOnIntegerOverflow=off  RndMeth=Floor
  MinMax1 : MinMax  Function=max  Inputs=2  InputSameDT=on  SaturateOnIntegerOverflow=on  ZeroCross=off
  MinMax2 : MinMax  Function=max  Inputs=2  InputSameDT=on  SaturateOnIntegerOverflow=on  ZeroCross=off
  MinMax3 : MinMax  Inputs=2  InputSameDT=on  SaturateOnIntegerOverflow=on  ZeroCross=off
  Product1 : Product  Inputs=/**  InputSameDT=on  OutDataTypeStr=Inherit: Same as first input
  Sat : $bdroot/Slink/Sat
  Sum : Sum  Inputs=++|  InputSameDT=on  OutDataTypeStr=Inherit: Same as first input
  Sum1 : Sum  Inputs=-|+  InputSameDT=on  OutDataTypeStr=Inherit: Same as first input
  Switch : Switch  Threshold=0.5  ZeroCross=off  SaturateOnIntegerOverflow=off
  Switch1 : Switch  Threshold=0.5  ZeroCross=off  SaturateOnIntegerOverflow=off
  Unit Delay : UnitDelay  InitialCondition=Zero  SampleTime=-1  HasFrameUpgradeWarning=on
      settings: AttributesFormatString=ic=%<X0>
  Unit Delay1 : UnitDelay  InitialCondition=Zero  SampleTime=-1  HasFrameUpgradeWarning=on
      settings: AttributesFormatString=ic=%<X0>
  Unit Delay2 : UnitDelay  InitialCondition=true  SampleTime=-1  HasFrameUpgradeWarning=on
      settings: AttributesFormatString=ic=%<X0>
  Output : Outport  VectorParamsAs1DForOutWhenUnconnected=off
  wires:
  Data Type Conversion/1 -> MinMax1/2, Product1/2
  Constant1/1 -> Data Type Conversion/1
  Unit Delay2/1 -> Switch1/2
  reset/1 -> Unit Delay2/1, Switch/2
  Product1/1 -> Sum/2
  Switch1/1 -> Product1/3, Unit Delay1/1
  Sum1/1 -> Switch1/1
  Unit Delay1/1 -> Switch1/3
  MinMax3/1 -> Sat/3
  MinMax2/1 -> Sat/2
  MinMax1/1 -> Product1/1
  C/1 -> MinMax1/1
  Sat/1 -> Unit Delay/1, Output/1
  Unit Delay/1 -> Sum/1
  Switch/1 -> Sat/1
  Sum/1 -> Switch/3
  B/1 -> MinMax2/2, MinMax3/2, Sum1/2
  A/1 -> MinMax3/1, MinMax2/1, Sum1/1, Switch/1

== system common_lib/Ctrl/Subsystem ==
  ClearCntrRqst : Inport
  Increment_Cntr : Inport  Port=2
  HWpd_Input : Inport  Port=3
  Constant15 : Constant  Value=uint32(1)
  Constant16 : Constant  Value=FALSE
  Constant17 : Constant  Value=MAX_UINT32
  Constant18 : Constant  Value=uint32(0)
  Constant19 : Constant  Value=uint32(0)
  Logical Operator9 : Logic  AllPortsSameDT=off
  Relational Operator6 : RelationalOperator  Operator=<  ZeroCross=off
  Sum4 : Sum  Inputs=|++  InputSameDT=on  OutDataTypeStr=Inherit: Same as first input
  Switch10 : Switch  Threshold=0.5  ZeroCross=off  SaturateOnIntegerOverflow=off
  Switch11 : Switch  Threshold=0.5  ZeroCross=off  SaturateOnIntegerOverflow=off
  Switch12 : Switch  Threshold=0.5  ZeroCross=off  SaturateOnIntegerOverflow=off
  Unit Delay8 : UnitDelay  InitialCondition=uint32(0)  SampleTime=-1  HasFrameUpgradeWarning=on
      settings: AttributesFormatString=ic=%<X0>
  Unit Delay9 : UnitDelay  InitialCondition=TRUE  SampleTime=-1  HasFrameUpgradeWarning=on
      settings: AttributesFormatString=ic=%<X0>
  CntrUpdate : Outport  VectorParamsAs1DForOutWhenUnconnected=off
  wires:
  Unit Delay8/1 -> Relational Operator6/1, Sum4/2
  Constant17/1 -> Relational Operator6/2
  Constant19/1 -> Switch12/1
  Switch10/1 -> Switch12/3
  Constant18/1 -> Switch11/3
  Constant15/1 -> Switch11/1
  Switch11/1 -> Sum4/1
  Sum4/1 -> Switch10/3
  Unit Delay9/1 -> Switch10/2
  Constant16/1 -> Unit Delay9/1
  Switch12/1 -> Unit Delay8/1, CntrUpdate/1
  Logical Operator9/1 -> Switch11/2
  Increment_Cntr/1 -> Logical Operator9/1
  Relational Operator6/1 -> Logical Operator9/2
  HWpd_Input/1 -> Switch10/1
  ClearCntrRqst/1 -> Switch12/2

== system common_lib/Ctrl/Trajectory ==
  note: Rate increment happens
      | even during reset
  note: Output - Final
  note: Start - Final
  note: Ignore the start_value
      | if it is moving away
      | from the final_value
  note: Reset if the previous value is further
      |                       away than the current start value
      | or if the final limit is smaller than the start limit
      | or if start is active
  note: Pick rate based on distance
      | from final
  note: Pick rate based on distance
      | from original start
  note: Start-CurrentStart
  note: Common Library::Control Structures::Trajectory Control
  start_value : Inport
  final_value : Inport  Port=2
  start_weight : Inport  Port=3
  stop_weight : Inport  Port=4
  start : Inport  Port=5
  Abs{,1,3..5} (5 alike) : Abs  ZeroCross=off  SaturateOnIntegerOverflow=off
  Constant1 : Constant  Value=MinusOne
  CurrentStart : Subsystem  TreatAsAtomicUnit=on
      settings: RTWSystemCode=Inline
  FinalRLim : Lookup  InputValues=FinalRLimIn  Table=FinalRLimOut  LookUpMeth=Interpolation-Use End Values  SaturateOnIntegerOverflow=off
  Logical Operator : Logic  Operator=OR  Inputs=3
  Logical Operator1 : Logic  Operator=OR
  MinMax3 : MinMax  Inputs=2  InputSameDT=on  SaturateOnIntegerOverflow=on  ZeroCross=off
  Relational Operator : RelationalOperator  Operator=<  ZeroCross=off
  Relational Operator1 : RelationalOperator  Operator=>  ZeroCross=off
  Relational Operator2 : RelationalOperator  ZeroCross=off
  Start : Subsystem  TreatAsAtomicUnit=on
      settings: RTWSystemCode=Inline
  StartRLim : Lookup  InputValues=StartRLimIn  Table=StartRLimOut  LookUpMeth=Interpolation-Use End Values  SaturateOnIntegerOverflow=off
  Sum1 : Sum  Inputs=-+  InputSameDT=on  OutDataTypeStr=Inherit: Same as first input
  Sum2 : Sum  Inputs=-+  InputSameDT=on  OutDataTypeStr=Inherit: Same as first input
  Sum3 : Sum  Inputs=+-  InputSameDT=on  OutDataTypeStr=Inherit: Same as first input
  Sum4 : Sum  Inputs=+-  InputSameDT=on  OutDataTypeStr=Inherit: Same as first input
  Sum6 : Sum  Inputs=+-  InputSameDT=on  OutDataTypeStr=Inherit: Same as first input
  Unit Delay1 : UnitDelay  InitialCondition=Zero  SampleTime=-1  HasFrameUpgradeWarning=on
      settings: AttributesFormatString=ic=%<X0>
  Unit Delay2 : UnitDelay  InitialCondition=Zero  SampleTime=-1  HasFrameUpgradeWarning=on
      settings: AttributesFormatString=ic=%<X0>
  Variable Rate Limiter w IC in feedback loop : Subsystem  mask(CL Variable Rate Limiter with Initial Condition){TimeStep=TimeStep, ic=Zero}
      mask prompts: TimeStep "Time Step"; ic "Initial Condition"
      mask help:
      | Variable rate limiter block with Initial Condiiton
      |
      | X(1) = input
      | X(2) = rise rate
      | X(3) = fall rate
      | X(4) = initial condition
      | X(5) = reset?
      |
      | Y(1) = output
      | NgEK, Inc.
      mask Help: web(which(['common_lib38.html']))
      mask Display:
      | patch([0.3 0.3 0.7 0.7], [0.35 0.65 0.65 0.35], [255/255 127/255 255/255])
      | 
      | plot([0 1],[0.5 0.5],[0.5 0.5],[0 1],[0 1],[0 1],[0.7 0.8 0.8],[0.8 0.8 0.7], [0.2 0.2 0.3],[0.3 0.2 0.2])
  transient_split3 : Product  InputSameDT=on  OutDataTypeStr=Inherit: Same as first input
  transient_split5 : Product  InputSameDT=on  OutDataTypeStr=Inherit: Same as first input
  transient_split6 : Product  InputSameDT=on  OutDataTypeStr=Inherit: Same as first input
  output : Outport  VectorParamsAs1DForOutWhenUnconnected=off
  wires:
  Abs5/1 -> Relational Operator2/1
  Sum4/1 -> Abs5/1
  Unit Delay2/1 -> Sum4/1
  Abs4/1 -> Relational Operator2/2
  Sum3/1 -> Abs4/1
  Relational Operator2/1 -> Logical Operator1/1
  Logical Operator1/1 -> CurrentStart/Enable
  CurrentStart/1(out) -> Start/1(in), Sum1/1, Unit Delay2/1, Variable Rate Limiter w IC in feedback loop/4(ic), Sum2/2
  Variable Rate Limiter w IC in feedback loop/1(output) -> Unit Delay1/1, output/1
  Relational Operator1/1 -> Logical Operator/1
  Abs3/1 -> Relational Operator1/1
  Sum6/1 -> Abs3/1
  Logical Operator/1 -> Variable Rate Limiter w IC in feedback loop/5(reset?)
  Unit Delay1/1 -> Sum6/1
  Relational Operator/1 -> Logical Operator/2
  transient_split5/1 -> Variable Rate Limiter w IC in feedback loop/3(fall rate)
  MinMax3/1 -> Variable Rate Limiter w IC in feedback loop/2(rise rate), transient_split5/1
  final_value/1 -> Sum4/2, Sum3/1, Variable Rate Limiter w IC in feedback loop/1(input), Sum6/2, Sum2/1
  transient_split6/1 -> Relational Operator/1, MinMax3/1
  FinalRLim/1 -> transient_split6/2
  Abs1/1 -> Relational Operator1/2, FinalRLim/1
  Sum2/1 -> Abs1/1
  Constant1/1 -> transient_split5/2
  stop_weight/1 -> transient_split6/1
  transient_split3/1 -> Relational Operator/2, MinMax3/2
  StartRLim/1 -> transient_split3/2
  Abs/1 -> StartRLim/1
  Sum1/1 -> Abs/1
  Start/1(out) -> Sum1/2
  start_weight/1 -> transient_split3/1
  start/1 -> Start/Enable, Logical Operator/3, Logical Operator1/2
  start_value/1 -> CurrentStart/1(in), Sum3/2

== system common_lib/Diag/CL MinMax Capture ==
  input : Inport
  hold? : Inport  Port=2
  reset? : Inport  Port=3
  Constant : Constant  Value=InitValue  SampleTime=-1
  Logical Operator : Logic  AllPortsSameDT=off
  Logical Operator1 : Logic  Operator=NOT  AllPortsSameDT=off
  Relational Operator : RelationalOperator  Operator=<  ZeroCross=off  InputSameDT=off
  Switch : Switch  Threshold=0.5  ZeroCross=off  SaturateOnIntegerOverflow=off  InputSameDT=off
  Switch1 : Switch  Threshold=0.5  ZeroCross=off  SaturateOnIntegerOverflow=off  InputSameDT=off
  Unit Delay : UnitDelay  InitialCondition=InitValue  SampleTime=-1  HasFrameUpgradeWarning=on
      settings: AttributesFormatString=ic=%<X0>
  Output Value : Outport  VectorParamsAs1DForOutWhenUnconnected=off
  wires:
  Constant/1 -> Switch/1
  reset?/1 -> Switch/2
  Switch1/1 -> Switch/3
  input/1 -> Switch1/1, Relational Operator/1  "Input"
  Relational Operator/1 -> Logical Operator/2  "Input past previous value"
  hold?/1 -> Logical Operator1/1  "Hold value"
  Logical Operator1/1 -> Logical Operator/1
  Logical Operator/1 -> Switch1/2  "New value"
  Switch/1 -> Unit Delay/1, Output Value/1
  Unit Delay/1 -> Switch1/3, Relational Operator/2  "Previous value"

== system common_lib/Diag/Command Feedback Test ==
  note: Common Library::Diagnostics::Command Feedback Test
  cmd : Inport
  fbk : Inport  Port=2
  tau : Inport  Port=3
  tau_lim : Inport  Port=4
  tau_time : Inport  Port=5
  error_lim : Inport  Port=6
  error_time : Inport  Port=7
  Enable : EnablePort  ZeroCross=off
  CommandFeedbackFaultLogicCore : Subsystem  TreatAsAtomicUnit=on  RTWFcnName=CFT
      settings: RTWFcnNameOpts=User specified  RTWFileNameOpts=Use function name
  Data Type Conversion{1..7} (7 alike) : DataTypeConversion  OutDataTypeStr=single  SaturateOnIntegerOverflow=off  RndMeth=Floor
  Signal Conversion : SignalConversion  ConversionOutput=Contiguous copy  OverrideOpt=on
  Min Value : Outport  VectorParamsAs1DForOutWhenUnconnected=off
  wires:
  cmd/1 -> Data Type Conversion7/1
  tau/1 -> Data Type Conversion5/1
  tau_lim/1 -> Data Type Conversion4/1
  tau_time/1 -> Data Type Conversion3/1
  error_lim/1 -> Data Type Conversion2/1
  CommandFeedbackFaultLogicCore/1(Min Value) -> Signal Conversion/1
  fbk/1 -> Data Type Conversion6/1
  error_time/1 -> Data Type Conversion1/1
  Signal Conversion/1 -> Min Value/1
  Data Type Conversion1/1 -> CommandFeedbackFaultLogicCore/7(error_time)
  Data Type Conversion2/1 -> CommandFeedbackFaultLogicCore/6(error_lim)
  Data Type Conversion3/1 -> CommandFeedbackFaultLogicCore/5(tau_time)
  Data Type Conversion4/1 -> CommandFeedbackFaultLogicCore/4(tau_lim)
  Data Type Conversion5/1 -> CommandFeedbackFaultLogicCore/3(tau)
  Data Type Conversion6/1 -> CommandFeedbackFaultLogicCore/2(fbk)
  Data Type Conversion7/1 -> CommandFeedbackFaultLogicCore/1(cmd)

== system common_lib/Diag/Fault Counter ==
  note: Common Library::Diagnostics::Fault Counter
  fl : Inport  OutDataTypeStr=boolean
  true_count : Inport  Port=2
  false_count : Inport  Port=3
  fc_level : Inport  Port=4
  reset : Inport  Port=5  OutDataTypeStr=boolean
  Compare To Zero : simulink/Logic and Bit Operations/Compare To Zero  relop=>  OutDataTypeStr=boolean  ZeroCross=off
  Constant : Constant  Value=true
  DTC : DataTypeConversion  OutDataTypeStr=boolean  SaturateOnIntegerOverflow=off  RndMeth=Floor
  DTC1 : DataTypeConversion  OutDataTypeStr=boolean  SaturateOnIntegerOverflow=off  RndMeth=Floor
  DTC3 : DataTypeConversion  OutDataTypeStr=int16  SaturateOnIntegerOverflow=off  RndMeth=Floor
  FaultCounter : Subsystem  RTWFcnName=FLTCNTR
      settings: RTWSystemCode=Inline  RTWFcnNameOpts=User specified  RTWFileNameOpts=Use function name
  Logical Operator : Logic  AllPortsSameDT=off  OutDataTypeStr=boolean
  Logical Operator1 : Logic  Operator=OR  AllPortsSameDT=off  OutDataTypeStr=boolean
  Signal Conversion : SignalConversion  ConversionOutput=Contiguous copy  OverrideOpt=on
  Unit Delay : UnitDelay  InitialCondition=ZERO  SampleTime=-1  HasFrameUpgradeWarning=on
      settings: AttributesFormatString=ic=%<X0>
  Unit Delay1 : UnitDelay  InitialCondition=false  SampleTime=-1  HasFrameUpgradeWarning=on
      settings: AttributesFormatString=ic=%<X0>
  inc switch : Switch  Criteria=u2 ~= 0  Threshold=0.5  ZeroCross=off  SaturateOnIntegerOverflow=off
  fc : Outport  VectorParamsAs1DForOutWhenUnconnected=off
  wires:
  FaultCounter/1(count) -> Unit Delay/1
  Unit Delay/1 -> FaultCounter/2(count_prev), Compare To Zero/1
  fc_level/1 -> DTC3/1
  reset/1 -> DTC1/1
  fl/1 -> DTC/1
  FaultCounter/2(fc) -> Signal Conversion/1
  Logical Operator/1 -> FaultCounter/Enable
  Constant/1 -> Unit Delay1/1
  Unit Delay1/1 -> Logical Operator/2
  Compare To Zero/1 -> Logical Operator1/1
  Logical Operator1/1 -> Logical Operator/1
  Signal Conversion/1 -> fc/1
  DTC/1 -> Logical Operator1/2, inc switch/2
  DTC1/1 -> FaultCounter/4(reset)
  DTC3/1 -> FaultCounter/3(fc_level)
  false_count/1 -> inc switch/3
  true_count/1 -> inc switch/1
  inc switch/1 -> FaultCounter/1(fl)
